simulink library "step2"  (R2018b)
settings: Solver=VariableStepAuto  StartTime=0.0  StopTime=10.0  RelTol=1e-3
settings Model: Creator=chris  LastModifiedBy=chris

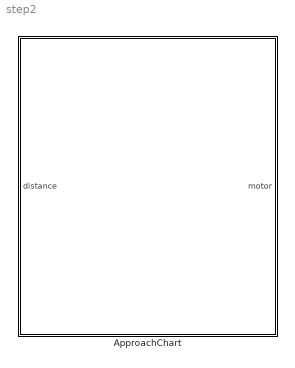
== system step2 ==
  "ApproachChart " : Stateflow chart  TreatAsAtomicUnit=on

== stateflow chart step2/ApproachChart  ==
  state Approach
    state Start
      entry: motor = 20
    state Wait
      entry: motor = 0
    state Exit
      entry: send(exitApproach)
    (default) -> Start
    Start -> Wait : [distance < stopDistance]
    Wait -> Exit : after(5, sec)
  state nextState
    % todo
    % go to next state
    % ??
  (default) -> Approach
  Approach -> nextState : exitApproach
  data: distance input; motor output; stopDistance constant double =20
  events: exitApproach local FUNCTION_CALL_EVENT
